simulink model "CountUpDown"  (R2021a)
settings: Solver=FixedStepDiscrete  StartTime=0.0  StopTime=10.0  RelTol=1e-3
settings Model: Creator=Dell  LastModifiedBy=Dell
settings OptimizationCC: DefaultParameterBehavior=Inlined  EnhancedBackFolding=on  PassReuseOutputArgsAs=Individual arguments  ZeroExternalMemoryAtStartup=off  ZeroInternalMemoryAtStartup=off  OptimizeBlockOrder=speed  DifferentSizesBufferReuse=on  OptimizationCustomize=off  EfficientTunableParamExpr=on
settings DebuggingCC: ParameterTunabilityLossMsg=error
settings SFSimCC: MATLABDynamicMemAlloc=off
settings RTWCC: SystemTargetFile=ert.tlc  GenCodeOnly=on  TemplateMakefile=ert_default_tmf  GenerateReport=on  IncludeHyperlinkInReport=on  LaunchReport=on  GenerateTraceInfo=on
settings CodeAppCC: ForceParamTrailComments=on  IgnoreCustomStorageClasses=off  OperatorAnnotations=on  SimulinkDataObjDesc=on  SFDataObjDesc=on  InsertBlockDesc=on
settings ERTTargetCC: TargetLangStandard=C99 (ISO)  GenerateSampleERTMain=on  InlinedParameterPlacement=NonHierarchical  ERTCustomFileTemplate=example_file_process.tlc

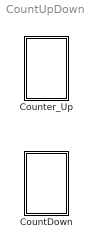
== system CountUpDown ==
  CountDown : Subsystem
  Counter_Up : Subsystem

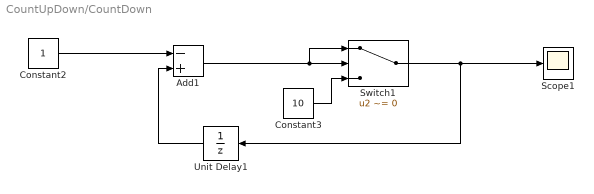
== system CountUpDown/CountDown ==
  Add1 : Sum  Inputs=-+  AccumDataTypeStr=uint8
  Constant2 : Constant  OutDataTypeStr=uint8
  Constant3 : Constant  Value=10
  Scope1 : Scope
  Switch1 : Switch  Criteria=u2 ~= 0  OutDataTypeStr=uint8
  Unit Delay1 : UnitDelay  InitialCondition=1  SampleTime=-1  HasFrameUpgradeWarning=on
  wires:
  Add1/1 -> Switch1/1, Switch1/2
  Unit Delay1/1 -> Add1/2
  Constant2/1 -> Add1/1
  Constant3/1 -> Switch1/3
  Switch1/1 -> Unit Delay1/1, Scope1/1

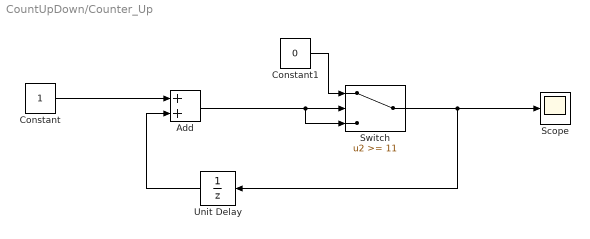
== system CountUpDown/Counter_Up ==
  Add : Sum
  Constant : Constant  OutDataTypeStr=uint8
  Constant1 : Constant  Value=0  OutDataTypeStr=uint8
  Scope : Scope
  Switch : Switch  Threshold=11  OutDataTypeStr=uint8
  Unit Delay : UnitDelay  SampleTime=-1  HasFrameUpgradeWarning=on
  wires:
  Constant1/1 -> Switch/1
  Constant/1 -> Add/1
  Add/1 -> Switch/3, Switch/2
  Switch/1 -> Unit Delay/1, Scope/1
  Unit Delay/1 -> Add/2
